simulink model "velocityEstimator"  (R2015b)
settings: Solver=FixedStepAuto  StartTime=0.0  StopTime=1000  FixedStep=0.1  RelTol=1e-3
libraries: robotlib x4, simulink x1
settings Model: Creator=sprinkle  LastModifiedBy=sprinkle

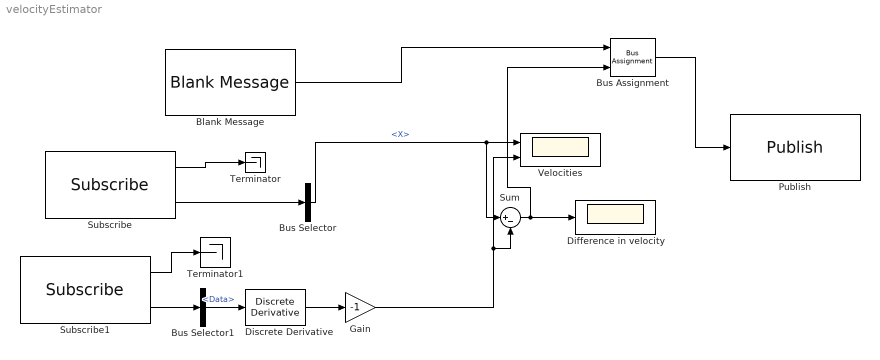
== system velocityEstimator ==
  Blank Message : robotlib/Blank Message  SourceLibraryInfo=This block requires Robotics System Toolbox  messageType=std_msgs/Float64  SampleTime=inf
  Bus Assignment : BusAssignment  AssignedSignals=Data
  Bus Selector : BusSelector  OutputSignals=Linear.X
  Bus Selector1 : BusSelector  OutputSignals=Data
  Difference in velocity : Scope
  Discrete Derivative : simulink/Discrete/Discrete Derivative  gainval=1.0  ICPrevScaledInput=0.0  InputProcessing=Inherited  OutMin=[]  OutMax=[]  OutDataType=fixdt(1, 16)  OutScaling=2^-10  DoSatur=off
  Gain : Gain  Gain=-1
  Publish : robotlib/Publish  SourceLibraryInfo=This block requires Robotics System Toolbox  topicSource=Specify your own  topic=/estimator/velocities  messageType=std_msgs/Float64  messageQueueLength=1
  Subscribe : robotlib/Subscribe  SourceLibraryInfo=This block requires Robotics System Toolbox  topicSource=Select from ROS network  topic=/azcar_sim/vel  messageType=geometry_msgs/Twist  sampleTime=-1  messageQueueLength=1
  Subscribe1 : robotlib/Subscribe  SourceLibraryInfo=This block requires Robotics System Toolbox  topicSource=Select from ROS network  topic=/DistanceEstimator/dist  messageType=std_msgs/Float32  sampleTime=-1  messageQueueLength=1
  Sum : Sum  Inputs=|+-
  Terminator : Terminator
  Terminator1 : Terminator
  Velocities : Scope  NumInputPorts=2
  wires:
  Subscribe/2 -> Bus Selector/1
  Subscribe/1 -> Terminator/1
  Bus Selector/1 -> Sum/1, Velocities/1  "<X>"
  Subscribe1/2 -> Bus Selector1/1
  Discrete Derivative/1 -> Gain/1
  Bus Selector1/1 -> Discrete Derivative/1  "<Data>"
  Sum/1 -> Bus Assignment/2, Difference in velocity/1
  Gain/1 -> Velocities/2, Sum/2
  Bus Assignment/1 -> Publish/1
  Subscribe1/1 -> Terminator1/1
  Blank Message/1 -> Bus Assignment/1
